simulink model "Modelo_nl222"  (R2015b)
settings: Solver=FixedStepDiscrete  StartTime=0  StopTime=15000  FixedStep=1  MaxStep=1  RelTol=1e-3
settings Model: Creator=gmiglio  LastModifiedBy=gmiglio

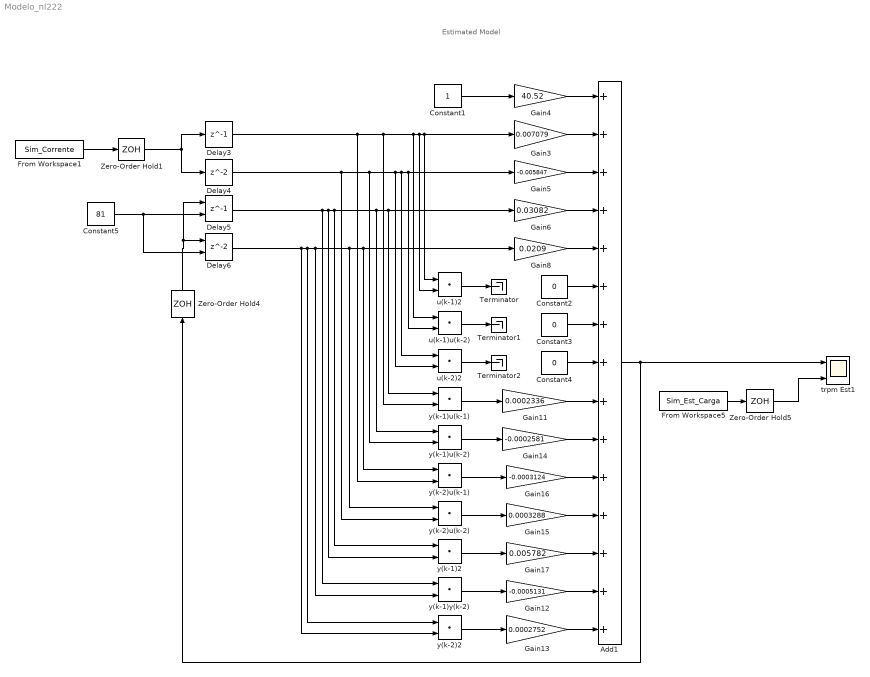
== system Modelo_nl222 ==
  note: Estimated Model
  Add1 : Sum  Inputs=+++++++++++++++
  Constant1 : Constant
  Constant2 : Constant  Value=0
  Constant3 : Constant  Value=0
  Constant4 : Constant  Value=0
  Constant5 : Constant  Value=81  SampleTime=-1
  Delay3 : Delay  DelayLength=1  InitialCondition=0
  Delay4 : Delay  InitialCondition=0
  Delay5 : Delay  DelayLength=1  InitialConditionSource=Input port  InitialCondition=81
      settings: InputPortMap=u0,p4
  Delay6 : Delay  InitialConditionSource=Input port  InitialCondition=81
      settings: InputPortMap=u0,p4
  From Workspace1 : FromWorkspace  VariableName=Sim_Corrente  SampleTime=0
  From Workspace5 : FromWorkspace  VariableName=Sim_Est_Carga  SampleTime=0
  Gain11 : Gain  Gain=0.0002336
  Gain12 : Gain  Gain=-0.0005131
  Gain13 : Gain  Gain=0.0002752
  Gain14 : Gain  Gain=-0.0002581
  Gain15 : Gain  Gain=0.0003288
  Gain16 : Gain  Gain=-0.0003124
  Gain17 : Gain  Gain=0.005782
  Gain3 : Gain  Gain=0.007079
  Gain4 : Gain  Gain=40.52
  Gain5 : Gain  Gain=-0.005847
  Gain6 : Gain  Gain=0.03082
  Gain8 : Gain  Gain=0.0209
  Terminator : Terminator
  Terminator1 : Terminator
  Terminator2 : Terminator
  Zero-Order Hold1 : ZeroOrderHold
  Zero-Order Hold4 : ZeroOrderHold
  Zero-Order Hold5 : ZeroOrderHold
  trpm Est1 : Scope  NumInputPorts=2
  u(k-1)2 : DotProduct  InputSameDT=on  OutDataTypeStr=Inherit: Inherit via internal rule
  u(k-1)u(k-2) : DotProduct  InputSameDT=on  OutDataTypeStr=Inherit: Inherit via internal rule
  u(k-2)2 : DotProduct  InputSameDT=on  OutDataTypeStr=Inherit: Inherit via internal rule
  y(k-1)2 : DotProduct  InputSameDT=on  OutDataTypeStr=Inherit: Inherit via internal rule
  y(k-1)u(k-1) : DotProduct  InputSameDT=on  OutDataTypeStr=Inherit: Inherit via internal rule
  y(k-1)u(k-2) : DotProduct  InputSameDT=on  OutDataTypeStr=Inherit: Inherit via internal rule
  y(k-1)y(k-2) : DotProduct  InputSameDT=on  OutDataTypeStr=Inherit: Inherit via internal rule
  y(k-2)2 : DotProduct  InputSameDT=on  OutDataTypeStr=Inherit: Inherit via internal rule
  y(k-2)u(k-1) : DotProduct  InputSameDT=on  OutDataTypeStr=Inherit: Inherit via internal rule
  y(k-2)u(k-2) : DotProduct  InputSameDT=on  OutDataTypeStr=Inherit: Inherit via internal rule
  wires:
  From Workspace1/1 -> Zero-Order Hold1/1
  Delay3/1 -> y(k-2)u(k-1)/2, y(k-1)u(k-1)/2, u(k-1)u(k-2)/1, u(k-1)2/2, u(k-1)2/1, Gain3/1
  Delay4/1 -> y(k-2)u(k-2)/2, y(k-1)u(k-2)/2, u(k-2)2/2, u(k-2)2/1, Gain5/1, u(k-1)u(k-2)/2
  Constant1/1 -> Gain4/1
  u(k-1)2/1 -> Terminator/1
  Delay5/1 -> y(k-1)y(k-2)/1, y(k-1)2/2, y(k-1)2/1, y(k-1)u(k-2)/1, Gain6/1, y(k-1)u(k-1)/1
  Delay6/1 -> y(k-2)2/2, y(k-2)2/1, y(k-1)y(k-2)/2, y(k-2)u(k-2)/1, Gain8/1, y(k-2)u(k-1)/1
  u(k-1)u(k-2)/1 -> Terminator1/1
  u(k-2)2/1 -> Terminator2/1
  y(k-1)u(k-1)/1 -> Gain11/1
  y(k-1)u(k-2)/1 -> Gain14/1
  y(k-2)u(k-1)/1 -> Gain16/1
  y(k-2)u(k-2)/1 -> Gain15/1
  y(k-1)2/1 -> Gain17/1
  y(k-1)y(k-2)/1 -> Gain12/1
  y(k-2)2/1 -> Gain13/1
  Zero-Order Hold1/1 -> Delay4/1, Delay3/1
  Gain4/1 -> Add1/1
  Gain3/1 -> Add1/2
  Gain5/1 -> Add1/3
  Gain6/1 -> Add1/4
  Gain8/1 -> Add1/5
  Constant2/1 -> Add1/6
  Constant3/1 -> Add1/7
  Constant4/1 -> Add1/8
  Gain11/1 -> Add1/9
  Gain14/1 -> Add1/10
  Gain16/1 -> Add1/11
  Gain15/1 -> Add1/12
  Gain17/1 -> Add1/13
  Gain12/1 -> Add1/14
  Gain13/1 -> Add1/15
  Add1/1 -> trpm Est1/1, Zero-Order Hold4/1
  From Workspace5/1 -> Zero-Order Hold5/1
  Zero-Order Hold5/1 -> trpm Est1/2
  Zero-Order Hold4/1 -> Delay5/1, Delay6/1
  Constant5/1 -> Delay6/2, Delay5/2
